simulink model "H_inf_control_2019b"  (R2019b)
settings: Solver=FixedStepAuto  StartTime=0  StopTime=10  FixedStep=0.002  RelTol=1e-3  EnableMultiTasking=on
PostLoadFcn:
  | qc_set_target_type(getConfigSet(bdroot, 'QUARC Default Target Configuration'));
values from neighbouring files (symbols this model uses):
  v_a_max = 10    [main.m]
undefined symbols (not defined in the file or in its folder): DiscIntNeverNeededParam, HIL, k2, Kr2, L22, qc_get_step_size, sigbuilder_block, sysest
libraries: simulink_extras x9, quarc_library x4, cstblocks x3
settings Model: SimulationMode=external  ExtModeTrigDuration=5000  Creator=CFulford  LastModifiedBy=AleFire
settings SolverCC: PositivePriorityOrder=on
settings DataIOCC: LimitDataPoints=on  SaveFormat=Array  SignalLoggingSaveFormat=ModelDataLogs  ReturnWorkspaceOutputs=off
settings OptimizationCC: ExpressionDepthLimit=2147483647  InitFltsAndDblsToZero=on  LifeSpan=inf
settings DebuggingCC: SaveWithParameterizedLinksMsg=none  UnderspecifiedInitializationDetection=Classic  MergeDetectMultiDrivingBlocksExec=none  SolverPrmCheckMsg=warning  MultiTaskDSMMsg=warning  MultiTaskCondExecSysMsg=none  FcnCallInpInsideContextMsg=warning  StateNameClashWarn=warning  SFUnexpectedBacktrackingDiag=warning  SFNoUnconditionalDefaultTransitionDiag=warning  SFExecutionAtInitializationDiag=none  ArithmeticOperatorsInVariantConditions=warning
settings HardwareCC: ProdBitPerPointer=32  ProdBitPerSizeT=32  ProdBitPerPtrDiffT=32  ProdLargestAtomicFloat=None  ProdIntDivRoundTo=Undefined  ProdEndianess=Unspecified  ProdWordSize=32  ProdHWDeviceType=32-bit Generic
settings ModelReferenceCC: PropagateSignalLabelsOutOfModel=off
settings SFSimCC: SimUseLocalCustomCode=off  CustomCodeUndefinedFunction=UseInterfaceOnly
settings RTWCC: Description=QUARC Win64 Target  SystemTargetFile=quarc_win64.tlc  TemplateMakefile=quarc_default_tmf  RTWUseLocalCustomCode=off
settings CodeAppCC: StateflowObjectComments=on
settings STFCustomTargetCC: TargetPreCompLibLocation=C:\PROGRA~3\QUARC\lib\2019b\win64\release  ConcurrentExecutionCompliant=on  CombineOutputUpdateFcns=on  CPPClassGenCompliant=on  SystemTargetFile=quarc_win64.tlc
settings GRTTargetCC: TargetPreCompLibLocation=C:\PROGRA~3\QUARC\lib\2019b\win64\release  TargetLangStandard=C89/C90 (ANSI)  ParMdlRefBuildCompliant=off  CompOptLevelCompliant=off  MatFileLogging=off  UseToolchainInfoCompliant=off  ExtMode=on  ExtModeMexFile=quarc_comm
settings ConfigComp: CovMetricSettings=dw  CovSaveCumulativeToWorkspaceVar=on  CovSaveSingleToWorkspaceVar=on  CovExternalEMLEnable=off  CovSFcnEnable=off

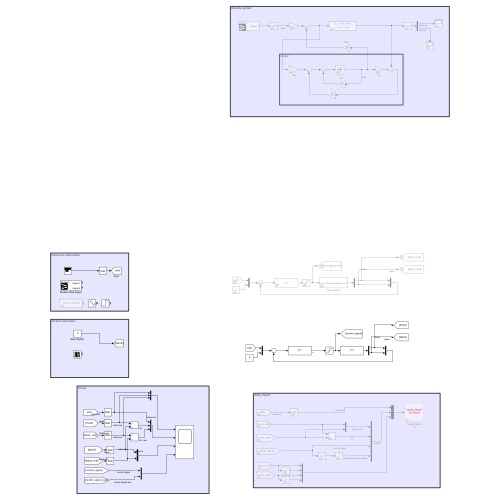
[thumbnail: Simulink's stored preview of the top-level diagram]
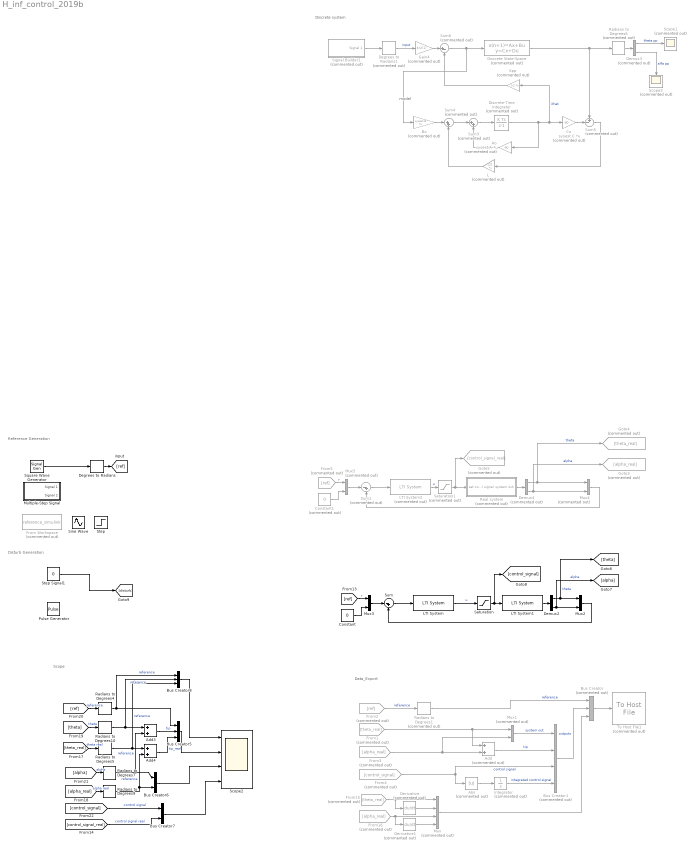
== system H_inf_control_2019b ==
  note: Reference Generation
  note: Disturb Generation
  note: Data_Export
  note: Discrete system
  note: model
  note: Scope
  Abs : Abs  Commented=on
  Add : Sum  Commented=on
  Add3 : Sum
  Add4 : Sum
  Ao : Gain  Commented=on  Gain=sysest.A  Multiplication=Matrix(K*u)
  Bo : Gain  Commented=on  Gain=sysest.B  Multiplication=Matrix(K*u)
  Bus Creator : BusCreator  Commented=on  Inputs=3
  Bus Creator1 : BusCreator  Commented=on  Inputs=4
  Bus Creator5 : BusCreator  Inputs=3
  Bus Creator6 : BusCreator  Inputs=2
  Bus Creator7 : BusCreator  Inputs=2
  Bus Creator8 : BusCreator  Inputs=3
  Co : Gain  Commented=on  Gain=sysest.C  Multiplication=Matrix(K*u)
  Constant : Constant  Value=0
  Constant1 : Constant  Commented=on  Value=0
  Degrees to Radians : simulink_extras/Transformations/Degrees to Radians
  Degrees to Radians1 : simulink_extras/Transformations/Degrees to Radians  Commented=on
  Demux2 : Demux  Outputs=2
  Demux3 : Demux  Commented=on  Outputs=2
  Demux4 : Demux  Commented=on  Outputs=2
  Derivative : Derivative  Commented=on
  Derivative1 : Derivative  Commented=on
  Discrete State-Space : DiscreteStateSpace  Commented=on  A=sysest.A  B=sysest.B  C=sysest.C  D=sysest.D  SampleTime=0.002
  Discrete-Time Integrator : DiscreteIntegrator  Commented=on  SampleTime=0.002  ICPrevOutput=DiscIntNeverNeededParam  ICPrevScaledInput=DiscIntNeverNeededParam
  From Workspace : FromWorkspace  Commented=on  VariableName=reference_simulink
  From1 : From  Commented=on  GotoTag=theta_real
  From15 : From  Commented=on  GotoTag=theta_real
  From16 : From  Commented=on  GotoTag=alpha_real
  From2 : From  Commented=on  GotoTag=ref
  From3 : From  Commented=on  GotoTag=alpha_real
  From4 : From  Commented=on  GotoTag=control_signal
  From5 : From  Commented=on  GotoTag=ref
  Gain4 : Gain  Commented=on  Gain=Kr2(1)
  Goto3 : Goto  Commented=on  GotoTag=alpha_real
  Goto4 : Goto  Commented=on  GotoTag=theta_real
  Goto5 : Goto  Commented=on  GotoTag=control_signal_real
  Integrator : Integrator  Commented=on
  Kpp : Gain  Commented=on  Gain=k2  Multiplication=Matrix(K*u)
  L : Gain  Commented=on  Gain=L22  Multiplication=Matrix(K*u)
  LTI System : cstblocks/LTI System  sys=K  IC=[]
  LTI System1 : cstblocks/LTI System  sys=sysest_ct  IC=[]
  LTI System2 : cstblocks/LTI System  Commented=on  sys=K  IC=[]
  Multiple-Step Signal : Subsystem  Tag=STV Subsys  LoadFcn=sigbuilder_block('load');  StartFcn=sigbuilder_block('start');  StopFcn=sigbuilder_block('stop');  ClipboardFcn=sigbuilder_block('clipboard');  mask(Sigbuilder block){tuvar=[0:10]}
      mask help: Simulink:masks:SigbuilderBlock_MD
      mask init:
      | if ~strcmp(get_param(bdroot(gcbh),'SimulationStatus'),'stopped') tuvar = sigbuilder_block('maskInit'); end
      settings: CopyFcn=sigbuilder_block('copy');  DeleteFcn=sigbuilder_block('delete');  ModelCloseFcn=sigbuilder_block('modelClose');  PreSaveFcn=sigbuilder_block('preSave');  PauseFcn=sigbuilder_block('pause');  ContinueFcn=sigbuilder_block('continue');  NameChangeFcn=sigbuilder_block('namechange');  OpenFcn=sigbuilder_block('open',[6 30 1428 681.75 ]);  CloseFcn=sigbuilder_block('close');
      mask Display: plot(0, 0, 100, 100,[2, 2, 32, 32, 2], [68, 8, 8, 68, 68],[32, 2], [38, 38], [32, 19, 2],[53, 60, 44], [32, 17, 17, 2],[16, 16, 31, 31]);txt = getActiveGroup(gcbh);text(2, 100, txt,'verticalAlignment', 'top');
  Mux : Mux  Commented=on
  Mux1 : Mux  Commented=on  Inputs=2
  Mux2 : Mux  Inputs=2
  Mux3 : Mux  Inputs=2
  Mux4 : Mux  Commented=on  Inputs=2
  Mux5 : Mux  Commented=on  Inputs=2
  Pulse Generator : DiscretePulseGenerator  PulseType=Time based  Period=10  PulseWidth=5
  Radians to Degrees1 : simulink_extras/Transformations/Radians to Degrees  Commented=on
  Radians to Degrees{4..5,7,9..10} (5 alike) : simulink_extras/Transformations/Radians to Degrees
  Radians to Degrees6 : simulink_extras/Transformations/Radians to Degrees  Commented=on
  Real system : Subsystem  Commented=on
  Saturation : Saturate  UpperLimit=v_a_max  LowerLimit=-v_a_max
  Saturation1 : Saturate  Commented=on  UpperLimit=v_a_max  LowerLimit=-v_a_max
  Scope1 : Scope  Commented=on
  Scope2 : Scope  NumInputPorts=4
  Scope3 : Scope  Commented=on
  Signal Builder1 : Subsystem  Tag=STV Subsys  Commented=on  LoadFcn=sigbuilder_block('load');  StartFcn=sigbuilder_block('start');  StopFcn=sigbuilder_block('stop');  ClipboardFcn=sigbuilder_block('clipboard');  mask(Sigbuilder block){tuvar=[0:10]}
      mask help: Simulink:masks:SigbuilderBlock_MD
      mask init:
      | if ~strcmp(get_param(bdroot(gcbh),'SimulationStatus'),'stopped') tuvar = sigbuilder_block('maskInit'); end
      settings: CopyFcn=sigbuilder_block('copy');  DeleteFcn=sigbuilder_block('delete');  ModelCloseFcn=sigbuilder_block('modelClose');  PreSaveFcn=sigbuilder_block('preSave');  PauseFcn=sigbuilder_block('pause');  ContinueFcn=sigbuilder_block('continue');  NameChangeFcn=sigbuilder_block('namechange');  OpenFcn=sigbuilder_block('open',[437.6 199.2 550.4 400 ]);  CloseFcn=sigbuilder_block('close');
      mask Display: plot(0, 0, 100, 100,[2, 2, 32, 32, 2], [68, 8, 8, 68, 68],[32, 2], [38, 38], [32, 19, 2],[53, 60, 44], [32, 17, 17, 2],[16, 16, 31, 31]);txt = getActiveGroup(gcbh);text(2, 100, txt,'verticalAlignment', 'top');
  Sine Wave : Sin  Amplitude=15  Frequency=4  SampleTime=0
  Square Wave Generator : SignalGenerator  WaveForm=square  Amplitude=20  Frequency=3  Units=rad/sec
  Step : Step  After=45  SampleTime=0
  Step Signal1 : Constant  Value=0
  Sum : Sum  Inputs=|-+
  Sum1 : Sum  Commented=on  Inputs=|-+
  Sum3 : Sum  Commented=on  Inputs=|++
  Sum4 : Sum  Commented=on  Inputs=|++
  Sum5 : Sum  Commented=on  Inputs=+-|
  Sum6 : Sum  Commented=on  Inputs=|+-
  To Host File1 : quarc_library/Sinks/To Host/To Host File  Commented=on  file_name=Sine tests\Sine_24_in_theta_alpha.mat  variable_name=data  decimation=1  sample_time=-1  file_format=MAT-file v.4  options=No header or footer  append=off  final_file_name=Sine tests\Sine_24_in_theta_alpha.mat  bitrate=2000000
  wires:
  From4/1 -> Abs/1, Bus Creator1/3  "control signal"
  Bus Creator1/1 -> Bus Creator/2  "outputs"
  From1/1 -> Add/1, Mux1/1
  Add/1 -> Bus Creator1/2  "tip"
  From2/1 -> Radians to Degrees1/1  "reference"
  Integrator/1 -> Bus Creator1/4  "integrated control signal"
  Bus Creator/1 -> To Host File1/1
  From3/1 -> Add/2, Mux1/2
  Degrees to Radians/1 -> [ref]
  Mux1/1 -> Bus Creator1/1  "system out"
  Sum5/1 -> L/1
  Demux3/1 -> Scope1/1  "theta pp"
  Sum6/1 -> Discrete State-Space/1, Bo/1
  L/1 -> Sum4/2
  Discrete State-Space/1 -> Radians to Degrees6/1, Sum5/1
  Sum4/1 -> Sum3/1
  Sum3/1 -> Discrete-Time Integrator/1
  Degrees to Radians1/1 -> Gain4/1  "input"
  Co/1 -> Sum5/2
  Demux3/2 -> Scope3/1  "alfa pp"
  Signal Builder1/1(Signal 1) -> Degrees to Radians1/1
  Kpp/1 -> Sum6/2
  Bo/1 -> Sum4/1
  Discrete-Time Integrator/1 -> Ao/1, Kpp/1, Co/1  "Xhat"
  Gain4/1 -> Sum6/1
  Ao/1 -> Sum3/2
  Radians to Degrees6/1 -> Demux3/1
  Radians to Degrees1/1 -> Bus Creator/1  "reference"
  Demux2/1 -> Mux2/1, [theta]  "theta"
  Demux2/2 -> Mux2/2, [alpha]  "alpha"
  Step Signal1/1 -> [disturb]
  Abs/1 -> Integrator/1
  From15/1 -> Derivative/1, Mux/1
  From16/1 -> Derivative1/1, Mux/3
  Mux/1 -> Bus Creator/3
  Derivative/1 -> Mux/2
  Derivative1/1 -> Mux/4
  LTI System1/1 -> Demux2/1
  Saturation/1 -> [control_signal], LTI System1/1
  Radians to Degrees9/1 -> Bus Creator6/2, Add4/2  "reference"
  Radians to Degrees10/1 -> Bus Creator8/2, Add3/1  "reference"
  [alpha] -> Radians to Degrees7/1  "alpha"
  [ref] -> Radians to Degrees4/1  "reference"
  [control_signal] -> Bus Creator7/1  "control signal"
  Add4/1 -> Bus Creator5/3  "tip_real"
  [theta_real] -> Radians to Degrees5/1  "theta real"
  [theta] -> Radians to Degrees10/1  "theta"
  Add3/1 -> Bus Creator5/2  "tip"
  [control_signal_real] -> Bus Creator7/2  "control signal real"
  Bus Creator6/1 -> Scope2/3
  Bus Creator8/1 -> Scope2/1
  Bus Creator7/1 -> Scope2/4
  Radians to Degrees7/1 -> Bus Creator6/1, Add3/2  "reference"
  Bus Creator5/1 -> Scope2/2
  Radians to Degrees4/1 -> Bus Creator8/1, Bus Creator5/1  "reference"
  [alpha_real] -> Radians to Degrees9/1  "alpha real"
  Radians to Degrees5/1 -> Bus Creator8/3, Add4/1  "reference"
  LTI System/1 -> Saturation/1  "u"
  Mux2/1 -> Sum/2
  [ref] -> Mux3/1  "r"
  Constant/1 -> Mux3/2
  Mux3/1 -> Sum/1
  Sum/1 -> LTI System/1
  Square Wave Generator/1 -> Degrees to Radians/1
  LTI System2/1 -> Saturation1/1  "u"
  Demux4/2 -> Goto3/1, Mux4/2  "alpha"
  Sum1/1 -> LTI System2/1
  Demux4/1 -> Goto4/1, Mux4/1  "theta"
  Constant1/1 -> Mux5/2
  Mux4/1 -> Sum1/2
  Mux5/1 -> Sum1/1
  From5/1 -> Mux5/1  "r"
  Saturation1/1 -> Goto5/1, Real system/1(sat control signal)
  Real system/1(system out) -> Demux4/1

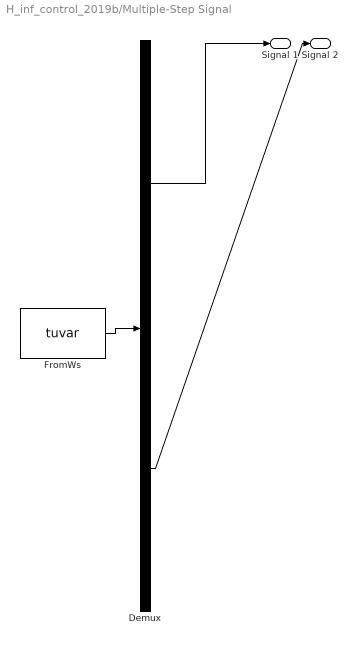
== system H_inf_control_2019b/Multiple-Step Signal ==
  Demux : Demux  Tag=STV Demux  Outputs=2
      settings: DisplayOption=none
  FromWs : FromWorkspace  Tag=STV FromWs  VariableName=tuvar
      SigBuilderData=|
      | common.afterFinalStr = 'Extrapolate'
      | common.sampleTime = 0
      | dataSet.timeRange = [0 10]
      | dataSet.name = 'Group 1'
      | sbobj.Groups.Name = 'Group 1'
      | sbobj.Groups.Signals(1).Name = 'Signal 1'
      | sbobj.Groups.Signals(1).XData = [0 1 1 3 3 7 7 8.5 8.5 10]
      | sbobj.Groups.Signals(1).YData = [0.005 0.005 40 40 -30 -30 0 0 23 23]
      | sbobj.Groups.Signals(2).Name = 'Signal 2'
      | sbobj.Groups.Signals(2).XData = [0 1 1 1.52 10]
      | sbobj.Groups.Signals(2).YData = [0 0 -40 -40 -40]
  Signal 1 : Outport  Tag=STV Outport
  Signal 2 : Outport  Tag=STV Outport  Port=2
  wires:
  Demux/1 -> Signal 1/1
  FromWs/1 -> Demux/1
  Demux/2 -> Signal 2/1

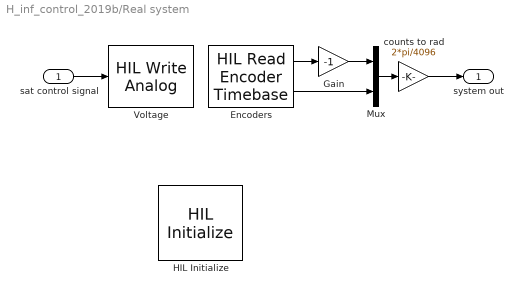
== system H_inf_control_2019b/Real system ==
  sat control signal : Inport
  Encoders : quarc_library/Data Acquisition/Generic/Timebases/HIL Read Encoder Timebase  object_name=HIL-1  clock=0  channels=[0:1]  samples_in_buffer=max(ceil(1/qc_get_step_size), 1)  active=on  vector_output=off  data_type_mode=Inherit via back propagation  data_type=double
  Gain : Gain  Gain=-1
  HIL Initialize : quarc_library/Data Acquisition/Generic/Configuration/HIL Initialize  Priority=-99  object_name=HIL-1  board_type=q2_usb  board_number=0  board_options=d0=digital;d1=digital;led=auto;update_rate=normal;decimation=1  exclusive=off  active=off  hardware_clocks=[0]  clock_modes=[]  initial_clock_frequencies=[]  set_clock_params_at_start=off  set_clock_params_at_switch_in=off  set_clock_frequencies_at_start=off  set_clock_frequencies_at_switch_in=off  analog_input_channels=[0:1]  analog_input_configurations=[]  analog_input_maximums=10  analog_input_minimums=-10  set_analog_input_params_at_start=on  set_analog_input_params_at_switch_in=off  analog_output_channels=[0:1]  analog_output_maximums=10  analog_output_minimums=-10  initial_analog_outputs=[0]  final_analog_outputs=[0]  watchdog_analog_outputs=0  set_analog_output_params_at_start=on  set_analog_output_params_at_switch_in=off  set_analog_outputs_at_start=on  set_analog_outputs_at_switch_in=off  set_analog_outputs_at_terminate=on  set_analog_outputs_at_switch_out=off  set_analog_outputs_on_watchdog=off  digital_input_channels=[]  digital_output_channels=[]  digital_output_configuration=[]  initial_digital_outputs=[1]  final_digital_outputs=[1]  watchdog_digital_outputs=[1]  set_digital_output_params_at_start=off  set_digital_output_params_at_switch_in=off  set_digital_outputs_at_start=on  set_digital_outputs_at_switch_in=off  set_digital_outputs_at_terminate=on  set_digital_outputs_at_switch_out=off  set_digital_outputs_on_watchdog=off  encoder_channels=[0:1]  quadrature=[4]  encoder_filter_frequency=[]  initial_encoder_counts=[0]  set_encoder_params_at_start=on  set_encoder_params_at_switch_in=off  set_encoder_counts_at_start=on  set_encoder_counts_at_switch_in=off  pwm_channels=[]  pwm_modes=[0]  pwm_frequency=1/0.020  pwm_configuration=[]  pwm_alignment=[]  pwm_polarity=[]  pwm_leading_deadband=[]  pwm_trailing_deadband=[]  initial_pwm_outputs=[0]  final_pwm_outputs=[0]  watchdog_pwm_outputs=[0]  set_pwm_params_at_start=on  set_pwm_params_at_switch_in=off  set_pwm_outputs_at_start=on  set_pwm_outputs_at_switch_in=off  set_pwm_outputs_at_terminate=on  set_pwm_outputs_at_switch_out=off  set_pwm_outputs_on_watchdog=off  other_output_channels=[]  initial_other_outputs=[]  final_other_outputs=[]  watchdog_other_outputs=[]  set_other_outputs_at_start=off  set_other_outputs_at_switch_in=off  set_other_outputs_at_terminate=off  set_other_outputs_at_switch_out=off  set_other_outputs_on_watchdog=off
  Mux : Mux  Inputs=2
  Voltage : quarc_library/Data Acquisition/Generic/Immediate I//O/HIL Write Analog  object_name=HIL-1  channels=0  sample_time=-1  active=off  vector_input=off
  counts to rad : Gain  Gain=2*pi/4096
  system out : Outport
  wires:
  sat control signal/1 -> Voltage/1
  Encoders/1 -> Gain/1
  Encoders/2 -> Mux/2
  Mux/1 -> counts to rad/1
  Gain/1 -> Mux/1
  counts to rad/1 -> system out/1

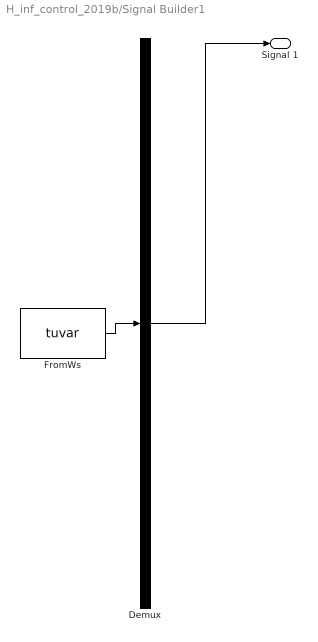
== system H_inf_control_2019b/Signal Builder1 ==
  Demux : Demux  Tag=STV Demux  Outputs=1
      settings: DisplayOption=none
  FromWs : FromWorkspace  Tag=STV FromWs  VariableName=tuvar
      SigBuilderData=|
      | common.afterFinalStr = 'Extrapolate'
      | common.sampleTime = 0
      | dataSet.timeRange = [0 10]
      | dataSet.name = 'Group 1'
      | sbobj.Groups.Name = 'Group 1'
      | sbobj.Groups.Signals.Name = 'Signal 1'
      | sbobj.Groups.Signals.XData = [0 1 1 3 3 5 5 7 7 8.5 8.5 10]
      | sbobj.Groups.Signals.YData = [0.005 0.005 40 40 15 15 -30 -30 0 0 23 23]
  Signal 1 : Outport  Tag=STV Outport
  wires:
  Demux/1 -> Signal 1/1
  FromWs/1 -> Demux/1
